simulink model "Simulate_CycleGAN"  (Simulink 10.2)
settings: Solver=ode45  StartTime=0.0  StopTime=30  RelTol=1e-3  EnableMultiTasking=on
libraries: slpidlib x16, fuzblock x4
settings Model: Creator=Administrator  LastModifiedBy=hunter
settings SolverCC: ZeroCrossControl=DisableAll
settings DataIOCC: LimitDataPoints=on
settings OptimizationCC: ExpressionDepthLimit=2147483647
settings DebuggingCC: SolverPrmCheckMsg=warning  StateNameClashWarn=warning

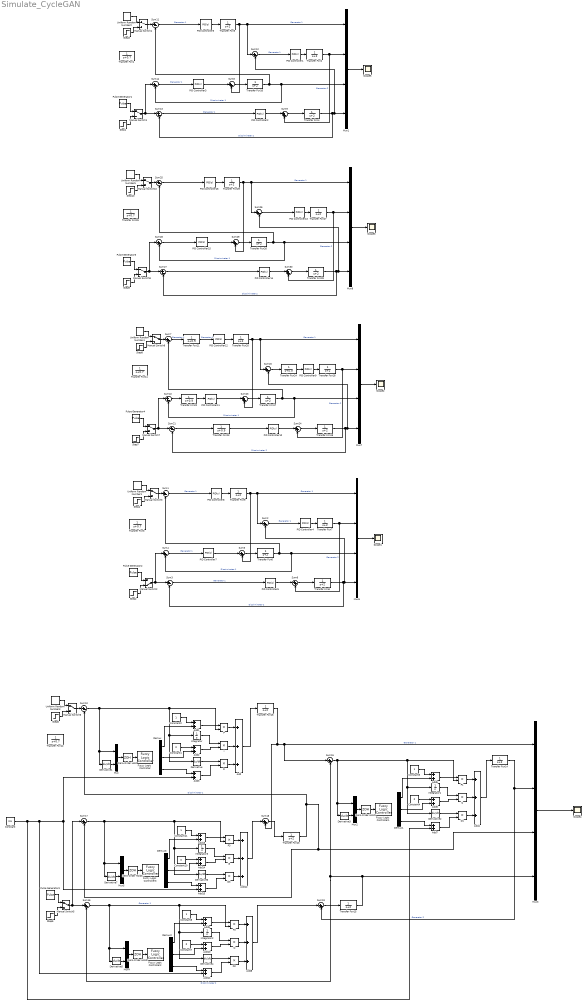
== system Simulate_CycleGAN ==
  Add{,4,8,12} (4 alike) : Sum  Inputs=+++
  Add{1..3,5..7,9..11,13..15} (12 alike) : Sum
  Constant : Constant  Value=0.5
  Constant{1,4,7,10} (4 alike) : Constant  Value=0
  Constant{2,5,8,11} (4 alike) : Constant
  D{,1..3} (4 alike) : Product
  Demux{,1..3} (4 alike) : Demux  Outputs=3
  Derivative{,1..7} (8 alike) : Derivative
  Fuzzy Logic  Controller{,1..3} (4 alike) : fuzblock/Fuzzy Logic  Controller  FIS="\"FuzzyPID002\""  OutputSampleNumber=101  DataType=double  FuzzifiedInputs=off  RuleFiringStrengths=off  RuleOutputs=off  AggregatedOutputs=off  SimulateUsing=Interpreted execution  OutOfRangeInputValueMessage=warning  NoRuleFiredMessage=warning  EmptyOutputFuzzySetMessage=warning
  I{,1..3} (4 alike) : Product
  Integrator{,1..3} (4 alike) : Integrator
  Manual Switch{1,3..10} (9 alike) : ManualSwitch
  Manual Switch2 : ManualSwitch  CurrentSetting=0
  Mux{,2,4..5} (4 alike) : Mux  Inputs=2
  Mux{1,3,6..8} (5 alike) : Mux
  P{,1..3} (4 alike) : Product
  PID Controller{1..3,5,9..12} (8 alike) : slpidlib/PID Controller  Controller=PID  Form=Parallel  TimeDomain=Continuous-time  UseExternalTs=off  SampleTime=-1  IntegratorMethod=Forward Euler  FilterMethod=Forward Euler  ControllerParametersSource=internal  P=1  I=0  D=0  UseFilter=on  N=100  TunerSelectOption=Transfer Function Based (PID Tuner App)  InitialConditionSource=internal  InitialConditionForIntegrator=0  InitialConditionForFilter=0  DifferentiatorICPrevScaledInput=0  ExternalReset=none  TrackingMode=off  Kt=1  LimitOutput=off  SatLimitsSource=internal  UpperSaturationLimit=inf  LowerSaturationLimit=-inf  LinearizeAsGain=on  AntiWindupMode=none  Kb=1  POutMin=[]  POutMax=[]  IOutMin=[]  IOutMax=[]  DOutMin=[]  DOutMax=[]  NOutMin=[]  NOutMax=[]  SumOutMin=[]  SumOutMax=[]  SaturationOutMin=[]  SaturationOutMax=[]  PParamMin=[]  PParamMax=[]  IParamMin=[]  IParamMax=[]  DParamMin=[]  DParamMax=[]  NParamMin=[]  NParamMax=[]  KbParamMin=[]  KbParamMax=[]  KtParamMin=[]  KtParamMax=[]  KbOutMin=[]  KbOutMax=[]  KtOutMin=[]  KtOutMax=[]  IntegratorOutMin=[]  IntegratorOutMax=[]  FilterOutMin=[]  FilterOutMax=[]  SumI1OutMin=[]  SumI1OutMax=[]  SumI2OutMin=[]  SumI2OutMax=[]  SumI3OutMin=[]  SumI3OutMax=[]  SumI4OutMin=[]  SumI4OutMax=[]  SumDOutMin=[]  SumDOutMax=[]  DifferentiatorOutMin=[]  DifferentiatorOutMax=[]  FilterDiffOutCoefMin=[]  FilterDiffOutCoefMax=[]  ReciprocalOutMin=[]  ReciprocalOutMax=[]  SumDenOutMin=[]  SumDenOutMax=[]  SumNumOutMin=[]  SumNumOutMax=[]  DivideOutMin=[]  DivideOutMax=[]  UdiffTsProdOutMin=[]  UdiffTsProdOutMax=[]  NTsProdOutMin=[]  NTsProdOutMax=[]  UintegralTsProdOutMin=[]  UintegralTsProdOutMax=[]  UngainTsProdOutMin=[]  UngainTsProdOutMax=[]  IntegratorContinuousStateAttributes=''  IntegratorStateMustResolveToSignalObject=off  IntegratorRTWStateStorageClass=Auto  FilterContinuousStateAttributes=''  FilterStateMustResolveToSignalObject=off  FilterRTWStateStorageClass=Auto  ParallelPVariant=InternalParameters  IdealPVariant=Disabled  IVariant=InternalParameters  DVariant=InternalParameters  IntegratorVariant=Continuous  SatVariant=Disabled  AWVariant=Passthrough  PCopyVariant=Disabled  TRVariant=Disabled  FdbkBlocksVariant=Forward  IdealPFdbkVariant=Disabled  SatFdbkVariant=Disabled  DerivativeFilterVariant=ContFilter  NVariant=InternalParameters  NCopyVariant=Disabled  FilterICVariant=InternalICsFilter  IntegratorICVariant=InternalICs  ExternalResetVariant=Disabled  TRSumVariant=Passthrough  SumFdbkVariant=Disabled  SumVariant=Sum_PID  TsampFilterVariant=InternalTs  TsampNgainVariant=Passthrough  TsampIntegralVariant=Passthrough  ExternalSaturationOutDataTypeStr=Inherit: Same as second input
  PID Controller{13..16} (4 alike) : slpidlib/PID Controller  Controller=PID  Form=Parallel  TimeDomain=Continuous-time  UseExternalTs=off  SampleTime=-1  IntegratorMethod=Forward Euler  FilterMethod=Forward Euler  ControllerParametersSource=internal  P=1  I=1  D=0  UseFilter=on  N=100  TunerSelectOption=Transfer Function Based (PID Tuner App)  InitialConditionSource=internal  InitialConditionForIntegrator=0  InitialConditionForFilter=0  DifferentiatorICPrevScaledInput=0  ExternalReset=none  TrackingMode=off  Kt=1  LimitOutput=off  SatLimitsSource=internal  UpperSaturationLimit=inf  LowerSaturationLimit=-inf  LinearizeAsGain=on  AntiWindupMode=none  Kb=1  POutMin=[]  POutMax=[]  IOutMin=[]  IOutMax=[]  DOutMin=[]  DOutMax=[]  NOutMin=[]  NOutMax=[]  SumOutMin=[]  SumOutMax=[]  SaturationOutMin=[]  SaturationOutMax=[]  PParamMin=[]  PParamMax=[]  IParamMin=[]  IParamMax=[]  DParamMin=[]  DParamMax=[]  NParamMin=[]  NParamMax=[]  KbParamMin=[]  KbParamMax=[]  KtParamMin=[]  KtParamMax=[]  KbOutMin=[]  KbOutMax=[]  KtOutMin=[]  KtOutMax=[]  IntegratorOutMin=[]  IntegratorOutMax=[]  FilterOutMin=[]  FilterOutMax=[]  SumI1OutMin=[]  SumI1OutMax=[]  SumI2OutMin=[]  SumI2OutMax=[]  SumI3OutMin=[]  SumI3OutMax=[]  SumI4OutMin=[]  SumI4OutMax=[]  SumDOutMin=[]  SumDOutMax=[]  DifferentiatorOutMin=[]  DifferentiatorOutMax=[]  FilterDiffOutCoefMin=[]  FilterDiffOutCoefMax=[]  ReciprocalOutMin=[]  ReciprocalOutMax=[]  SumDenOutMin=[]  SumDenOutMax=[]  SumNumOutMin=[]  SumNumOutMax=[]  DivideOutMin=[]  DivideOutMax=[]  UdiffTsProdOutMin=[]  UdiffTsProdOutMax=[]  NTsProdOutMin=[]  NTsProdOutMax=[]  UintegralTsProdOutMin=[]  UintegralTsProdOutMax=[]  UngainTsProdOutMin=[]  UngainTsProdOutMax=[]  IntegratorContinuousStateAttributes=''  IntegratorStateMustResolveToSignalObject=off  IntegratorRTWStateStorageClass=Auto  FilterContinuousStateAttributes=''  FilterStateMustResolveToSignalObject=off  FilterRTWStateStorageClass=Auto  ParallelPVariant=InternalParameters  IdealPVariant=Disabled  IVariant=InternalParameters  DVariant=InternalParameters  IntegratorVariant=Continuous  SatVariant=Disabled  AWVariant=Passthrough  PCopyVariant=Disabled  TRVariant=Disabled  FdbkBlocksVariant=Forward  IdealPFdbkVariant=Disabled  SatFdbkVariant=Disabled  DerivativeFilterVariant=ContFilter  NVariant=InternalParameters  NCopyVariant=Disabled  FilterICVariant=InternalICsFilter  IntegratorICVariant=InternalICs  ExternalResetVariant=Disabled  TRSumVariant=Passthrough  SumFdbkVariant=Disabled  SumVariant=Sum_PID  TsampFilterVariant=InternalTs  TsampNgainVariant=Passthrough  TsampIntegralVariant=Passthrough  ExternalSaturationOutDataTypeStr=Inherit: Same as second input
  PID Controller{4,6..8} (4 alike) : slpidlib/PID Controller  Controller=PID  Form=Parallel  TimeDomain=Continuous-time  UseExternalTs=off  SampleTime=-1  IntegratorMethod=Forward Euler  FilterMethod=Forward Euler  ControllerParametersSource=internal  P=1  I=1  D=0.5  UseFilter=on  N=100  TunerSelectOption=Transfer Function Based (PID Tuner App)  InitialConditionSource=internal  InitialConditionForIntegrator=0  InitialConditionForFilter=0  DifferentiatorICPrevScaledInput=0  ExternalReset=none  TrackingMode=off  Kt=1  LimitOutput=off  SatLimitsSource=internal  UpperSaturationLimit=inf  LowerSaturationLimit=-inf  LinearizeAsGain=on  AntiWindupMode=none  Kb=1  POutMin=[]  POutMax=[]  IOutMin=[]  IOutMax=[]  DOutMin=[]  DOutMax=[]  NOutMin=[]  NOutMax=[]  SumOutMin=[]  SumOutMax=[]  SaturationOutMin=[]  SaturationOutMax=[]  PParamMin=[]  PParamMax=[]  IParamMin=[]  IParamMax=[]  DParamMin=[]  DParamMax=[]  NParamMin=[]  NParamMax=[]  KbParamMin=[]  KbParamMax=[]  KtParamMin=[]  KtParamMax=[]  KbOutMin=[]  KbOutMax=[]  KtOutMin=[]  KtOutMax=[]  IntegratorOutMin=[]  IntegratorOutMax=[]  FilterOutMin=[]  FilterOutMax=[]  SumI1OutMin=[]  SumI1OutMax=[]  SumI2OutMin=[]  SumI2OutMax=[]  SumI3OutMin=[]  SumI3OutMax=[]  SumI4OutMin=[]  SumI4OutMax=[]  SumDOutMin=[]  SumDOutMax=[]  DifferentiatorOutMin=[]  DifferentiatorOutMax=[]  FilterDiffOutCoefMin=[]  FilterDiffOutCoefMax=[]  ReciprocalOutMin=[]  ReciprocalOutMax=[]  SumDenOutMin=[]  SumDenOutMax=[]  SumNumOutMin=[]  SumNumOutMax=[]  DivideOutMin=[]  DivideOutMax=[]  UdiffTsProdOutMin=[]  UdiffTsProdOutMax=[]  NTsProdOutMin=[]  NTsProdOutMax=[]  UintegralTsProdOutMin=[]  UintegralTsProdOutMax=[]  UngainTsProdOutMin=[]  UngainTsProdOutMax=[]  IntegratorContinuousStateAttributes=''  IntegratorStateMustResolveToSignalObject=off  IntegratorRTWStateStorageClass=Auto  FilterContinuousStateAttributes=''  FilterStateMustResolveToSignalObject=off  FilterRTWStateStorageClass=Auto  ParallelPVariant=InternalParameters  IdealPVariant=Disabled  IVariant=InternalParameters  DVariant=InternalParameters  IntegratorVariant=Continuous  SatVariant=Disabled  AWVariant=Passthrough  PCopyVariant=Disabled  TRVariant=Disabled  FdbkBlocksVariant=Forward  IdealPFdbkVariant=Disabled  SatFdbkVariant=Disabled  DerivativeFilterVariant=ContFilter  NVariant=InternalParameters  NCopyVariant=Disabled  FilterICVariant=InternalICsFilter  IntegratorICVariant=InternalICs  ExternalResetVariant=Disabled  TRSumVariant=Passthrough  SumFdbkVariant=Disabled  SumVariant=Sum_PID  TsampFilterVariant=InternalTs  TsampNgainVariant=Passthrough  TsampIntegralVariant=Passthrough  ExternalSaturationOutDataTypeStr=Inherit: Same as second input
  Pulse Generator{1..5} (5 alike) : DiscretePulseGenerator  PulseType=Time based  Period=5  PulseWidth=50
  Scope{1..5} (5 alike) : Scope
  Step{1..2,5,7,9} (5 alike) : Step  Time=0  SampleTime=0
  Step{3..4,6,8,10} (5 alike) : Step  Time=10  SampleTime=0
  Sum{1..4,7,10..17,20..22,25..28} (20 alike) : Sum  Inputs=|+-
  Sum{5..6,8..9,18..19,23..24,29..30} (10 alike) : Sum  Inputs=|++
  Transfer Fcn{1,3,11..12,25} (5 alike) : TransferFcn  Denominator=[1 0.7]
  Transfer Fcn{2,4..10,13..20,26..29} (20 alike) : TransferFcn  Denominator=[1 2]
  Transfer Fcn{21..24} (4 alike) : TransferFcn  Denominator=[1 0.9]
  Uniform Random Number{1..5} (5 alike) : UniformRandomNumber  SampleTime=0.1
  Zero-Order Hold{,1..3} (4 alike) : ZeroOrderHold
  wires:
  Pulse Generator1/1 -> Manual Switch1/1
  Sum9/1 -> Transfer Fcn4/1
  Transfer Fcn10/1 -> Mux1/3, Sum14/2, Sum11/2  "Discriminater 1"
  Sum13/1 -> PID Controller2/1  "Generator 1"
  Manual Switch4/1 -> Sum11/1
  Sum12/1 -> PID Controller1/1  "Generator 1"
  PID Controller3/1 -> Sum8/1
  Transfer Fcn2/1 -> Sum9/2, Mux1/2  "Generator 2"
  Sum8/1 -> Transfer Fcn10/1
  Sum14/1 -> PID Controller3/1  "Generator 1"
  Step3/1 -> Manual Switch4/2
  Step1/1 -> Manual Switch1/2
  PID Controller1/1 -> Transfer Fcn2/1
  Sum11/1 -> PID Controller5/1  "Generator 1"
  Manual Switch1/1 -> Sum13/1, Sum14/1
  Transfer Fcn4/1 -> Sum12/2, Mux1/4, Sum13/2  "Discriminater 2"
  Uniform Random Number2/1 -> Manual Switch4/1
  PID Controller2/1 -> Sum9/1
  Transfer Fcn5/1 -> Sum8/2, Mux1/1, Sum12/1  "Generator 1"
  Mux1/1 -> Scope5/1
  PID Controller5/1 -> Transfer Fcn5/1
  Integrator/1 -> I/1
  Derivative1/1 -> Mux/2
  Add3/1 -> D/2
  I/1 -> Add/2
  Constant1/1 -> Add2/1
  Add2/1 -> I/2
  Mux/1 -> Zero-Order Hold/1
  Add/1 -> Transfer Fcn16/1
  Constant2/1 -> Add1/1
  Sum10/1 -> Derivative/1, Integrator/1, P/2, Derivative1/1, Mux/1
  Derivative/1 -> D/1
  P/1 -> Add/1
  Demux/1 -> Add1/2
  Add1/1 -> P/1
  Demux/3 -> Add3/1
  Demux/2 -> Add2/2
  D/1 -> Add/3
  Transfer Fcn16/1 -> Sum18/2, Sum15/1, Mux3/1  "Generator 1"
  Mux3/1 -> Scope4/1
  Uniform Random Number3/1 -> Manual Switch6/1
  Step6/1 -> Manual Switch6/2
  Manual Switch5/1 -> Sum16/1, Sum17/1
  Step5/1 -> Manual Switch5/2
  Sum18/1 -> Transfer Fcn13/1
  Transfer Fcn14/1 -> Mux3/2, Sum19/2  "Generator 2"
  Transfer Fcn15/1 -> Mux3/4, Sum16/2, Sum15/2  "Discriminater 2"
  Sum19/1 -> Transfer Fcn15/1
  Manual Switch6/1 -> Sum10/1
  Transfer Fcn13/1 -> Sum10/2, Mux3/3, Sum17/2  "Discriminater 1"
  Pulse Generator3/1 -> Manual Switch5/1
  Zero-Order Hold/1 -> Fuzzy Logic  Controller/1
  D1/1 -> Add4/3
  Demux1/2 -> Add6/2
  Demux1/3 -> Add7/1
  Add5/1 -> P1/1
  Demux1/1 -> Add5/2
  Derivative2/1 -> D1/1
  Sum15/1 -> Derivative2/1, Integrator1/1, P1/2, Derivative3/1, Mux2/1
  Mux2/1 -> Zero-Order Hold1/1
  Constant5/1 -> Add5/1
  P1/1 -> Add4/1
  Add4/1 -> Transfer Fcn14/1
  Constant4/1 -> Add6/1
  I1/1 -> Add4/2
  Add7/1 -> D1/2
  Integrator1/1 -> I1/1
  Derivative3/1 -> Mux2/2
  Add6/1 -> I1/2
  D2/1 -> Add8/3
  Demux2/2 -> Add10/2
  Demux2/3 -> Add11/1
  Add9/1 -> P2/1
  Demux2/1 -> Add9/2
  Derivative4/1 -> D2/1
  Mux4/1 -> Zero-Order Hold2/1
  Constant8/1 -> Add9/1
  P2/1 -> Add8/1
  Add8/1 -> Sum19/1
  Constant7/1 -> Add10/1
  I2/1 -> Add8/2
  Add11/1 -> D2/2
  Integrator2/1 -> I2/1
  Derivative5/1 -> Mux4/2
  Add10/1 -> I2/2
  Sum16/1 -> Derivative4/1, Integrator2/1, P2/2, Derivative5/1, Mux4/1  "Generator 1"
  D3/1 -> Add12/3
  Demux3/2 -> Add14/2
  Demux3/3 -> Add15/1
  Add13/1 -> P3/1
  Demux3/1 -> Add13/2
  Derivative6/1 -> D3/1
  Sum17/1 -> Derivative6/1, Integrator3/1, P3/2, Derivative7/1, Mux5/1
  Mux5/1 -> Zero-Order Hold3/1
  Constant11/1 -> Add13/1
  P3/1 -> Add12/1
  Add12/1 -> Sum18/1
  Constant10/1 -> Add14/1
  I3/1 -> Add12/2
  Add15/1 -> D3/2
  Integrator3/1 -> I3/1
  Derivative7/1 -> Mux5/2
  Add14/1 -> I3/2
  Zero-Order Hold1/1 -> Fuzzy Logic  Controller1/1
  Constant/1 -> Add15/2, Add3/2, Add11/2, Add7/2
  Zero-Order Hold3/1 -> Fuzzy Logic  Controller3/1
  Zero-Order Hold2/1 -> Fuzzy Logic  Controller2/1
  Transfer Fcn9/1 -> Sum5/2, Mux6/1, Sum2/1  "Generator 1"
  Mux6/1 -> Scope1/1
  PID Controller8/1 -> Transfer Fcn9/1
  PID Controller6/1 -> Sum6/1
  Uniform Random Number1/1 -> Manual Switch3/1
  Sum1/1 -> PID Controller8/1  "Generator 1"
  PID Controller4/1 -> Transfer Fcn7/1
  Step4/1 -> Manual Switch3/2
  Manual Switch2/1 -> Sum3/1, Sum4/1
  Step2/1 -> Manual Switch2/2
  Sum4/1 -> PID Controller7/1  "Generator 1"
  PID Controller7/1 -> Sum5/1
  Sum5/1 -> Transfer Fcn6/1
  Transfer Fcn7/1 -> Sum6/2, Mux6/2  "Generator 2"
  Transfer Fcn8/1 -> Sum2/2, Mux6/4, Sum3/2  "Discriminater 2"
  Sum6/1 -> Transfer Fcn8/1
  Sum3/1 -> PID Controller6/1  "Generator 1"
  Manual Switch3/1 -> Sum1/1
  Transfer Fcn6/1 -> Mux6/3, Sum4/2, Sum1/2  "Discriminater 1"
  Pulse Generator2/1 -> Manual Switch2/1
  Sum2/1 -> PID Controller4/1  "Generator 1"
  Transfer Fcn20/1 -> Sum23/2, Mux7/1, Sum20/1  "Generator 1"
  Mux7/1 -> Scope2/1
  PID Controller12/1 -> Transfer Fcn20/1
  PID Controller10/1 -> Sum24/1
  Uniform Random Number4/1 -> Manual Switch8/1
  PID Controller9/1 -> Transfer Fcn18/1
  Step8/1 -> Manual Switch8/2
  Manual Switch7/1 -> Sum21/1, Sum22/1
  Step7/1 -> Manual Switch7/2
  PID Controller11/1 -> Sum23/1
  Sum23/1 -> Transfer Fcn17/1
  Transfer Fcn18/1 -> Sum24/2, Mux7/2  "Generator 2"
  Transfer Fcn19/1 -> Sum20/2, Mux7/4, Sum21/2  "Discriminater 2"
  Sum24/1 -> Transfer Fcn19/1
  Manual Switch8/1 -> Sum7/1
  Transfer Fcn17/1 -> Mux7/3, Sum22/2, Sum7/2  "Discriminater 1"
  Pulse Generator4/1 -> Manual Switch7/1
  Sum7/1 -> Transfer Fcn21/1  "Generator 1"
  Transfer Fcn21/1 -> PID Controller12/1  "Generator 1"
  Transfer Fcn22/1 -> PID Controller11/1
  Sum22/1 -> Transfer Fcn22/1
  Sum21/1 -> Transfer Fcn23/1
  Transfer Fcn23/1 -> PID Controller10/1
  Transfer Fcn24/1 -> PID Controller9/1
  Sum20/1 -> Transfer Fcn24/1
  Transfer Fcn29/1 -> Sum29/2, Mux8/1, Sum26/1  "Generator 1"
  Mux8/1 -> Scope3/1
  PID Controller16/1 -> Transfer Fcn29/1
  PID Controller14/1 -> Sum30/1
  Uniform Random Number5/1 -> Manual Switch10/1
  Sum25/1 -> PID Controller16/1
  PID Controller13/1 -> Transfer Fcn27/1
  Step10/1 -> Manual Switch10/2
  Manual Switch9/1 -> Sum27/1, Sum28/1
  Step9/1 -> Manual Switch9/2
  Sum28/1 -> PID Controller15/1
  PID Controller15/1 -> Sum29/1
  Sum29/1 -> Transfer Fcn26/1
  Transfer Fcn27/1 -> Sum30/2, Mux8/2  "Generator 2"
  Transfer Fcn28/1 -> Sum26/2, Mux8/4, Sum27/2  "Discriminater 2"
  Sum30/1 -> Transfer Fcn28/1
  Sum27/1 -> PID Controller14/1
  Manual Switch10/1 -> Sum25/1
  Transfer Fcn26/1 -> Mux8/3, Sum28/2, Sum25/2  "Discriminater 1"
  Pulse Generator5/1 -> Manual Switch9/1
  Sum26/1 -> PID Controller13/1
